simulink subsystem "Pumpstation_Controller"  (R2022b)
settings: Solver=VariableStepAuto  StartTime=0.0  StopTime=10.0  RelTol=1e-3
model mask{Speedlimit_Upper=95, Speedlimit_Lower=65, TotalPumps=3, Kp=0, Ki=0}
  mask prompts: Speedlimit_Upper "Upper limit on pump speed"; Speedlimit_Lower "Lower limit on pump speed"; TotalPumps "Total number of pumps"
libraries: slpidlib x1
settings Model: Creator=Fie  LastModifiedBy=pppc

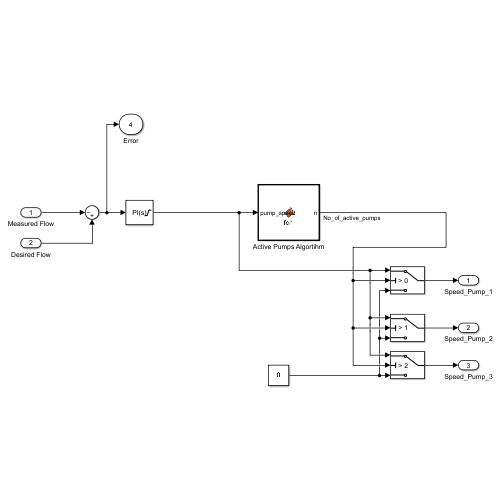
[thumbnail: Simulink's stored preview of the top-level diagram]
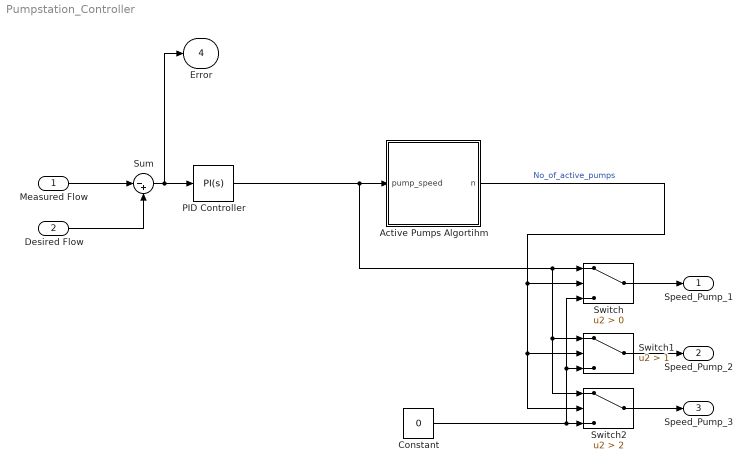
== system Pumpstation_Controller ==
  Measured Flow : Inport
  Desired Flow : Inport  Port=2
  Active Pumps Algortihm : MATLAB Function  TreatAsAtomicUnit=on  SystemSampleTime=10
  Constant : Constant  Value=0
  PID Controller : slpidlib/PID Controller  Controller=PI  Form=Parallel  TimeDomain=Continuous-time  UseExternalTs=off  SampleTime=-1  IntegratorMethod=Forward Euler  FilterMethod=Forward Euler  ControllerParametersSource=internal  P=Kp  I=Ki  UseKiTs=off  D=0  N=100  UseFilter=on  TunerSelectOption=Transfer Function Based (PID Tuner App)  InitialConditionSource=internal  InitialConditionForIntegrator=40  InitialConditionForFilter=0  DifferentiatorICPrevScaledInput=0  ExternalReset=none  TrackingMode=off  Kt=1  LimitOutput=on  SatLimitsSource=internal  UpperSaturationLimit=100  LowerSaturationLimit=0  LinearizeAsGain=on  AntiWindupMode=back-calculation  Kb=1  LimitIntegrator=off  UpperIntegratorSaturationLimit=inf  LowerIntegratorSaturationLimit=-inf  POutMin=[]  POutMax=[]  IOutMin=[]  IOutMax=[]  DOutMin=[]  DOutMax=[]  NOutMin=[]  NOutMax=[]  SumOutMin=[]  SumOutMax=[]  SaturationOutMin=[]  SaturationOutMax=[]  PParamMin=[]  PParamMax=[]  IParamMin=[]  IParamMax=[]  DParamMin=[]  DParamMax=[]  NParamMin=[]  NParamMax=[]  KbParamMin=[]  KbParamMax=[]  KtParamMin=[]  KtParamMax=[]  KbOutMin=[]  KbOutMax=[]  KtOutMin=[]  KtOutMax=[]  IntegratorOutMin=[]  IntegratorOutMax=[]  FilterOutMin=[]  FilterOutMax=[]  SumI1OutMin=[]  SumI1OutMax=[]  SumI2OutMin=[]  SumI2OutMax=[]  SumI3OutMin=[]  SumI3OutMax=[]  SumI4OutMin=[]  SumI4OutMax=[]  SumDOutMin=[]  SumDOutMax=[]  DifferentiatorOutMin=[]  DifferentiatorOutMax=[]  FilterDiffOutCoefMin=[]  FilterDiffOutCoefMax=[]  ReciprocalOutMin=[]  ReciprocalOutMax=[]  SumDenOutMin=[]  SumDenOutMax=[]  SumNumOutMin=[]  SumNumOutMax=[]  DivideOutMin=[]  DivideOutMax=[]  UdiffTsProdOutMin=[]  UdiffTsProdOutMax=[]  NTsProdOutMin=[]  NTsProdOutMax=[]  UintegralTsProdOutMin=[]  UintegralTsProdOutMax=[]  UngainTsProdOutMin=[]  UngainTsProdOutMax=[]  ClampingZeroOutDataTypeStr=Inherit: Inherit via back propagation  ClampingZeroOutMin=[]  ClampingZeroOutMax=[]  FilterDenConstantOutDataTypeStr=Inherit: Inherit via back propagation  FilterDenConstantOutMin=[]  FilterDenConstantOutMax=[]  PCopyOutDataTypeStr=Inherit: Inherit via back propagation  PCopyOutMin=[]  PCopyOutMax=[]  NCopyOutDataTypeStr=Inherit: Inherit via back propagation  NCopyOutMin=[]  NCopyOutMax=[]  IntegratorContinuousStateAttributes=''  IntegratorStateMustResolveToSignalObject=off  IntegratorRTWStateStorageClass=Auto  FilterContinuousStateAttributes=''  FilterStateMustResolveToSignalObject=off  FilterRTWStateStorageClass=Auto  ParallelPVariant=InternalParameters  IdealPVariant=Disabled  IVariant=InternalParameters  DVariant=Disabled  IntegratorVariant=Continuous  SatVariant=Enabled  AWVariant=BackCalculation  PCopyVariant=Disabled  TRVariant=Disabled  FdbkBlocksVariant=Forward  IdealPFdbkVariant=Disabled  SatFdbkVariant=Disabled  DerivativeFilterVariant=Disabled  NVariant=Disabled  NCopyVariant=Disabled_SignalSpec  FilterICVariant=Disabled  IntegratorICVariant=InternalICs  ExternalResetVariant=Disabled  TRSumVariant=Passthrough  SumFdbkVariant=Disabled  SumVariant=Sum_PI  TsampFilterVariant=InternalTs  TsampNgainVariant=Passthrough  TsampIntegralVariant=Passthrough  ExternalSaturationOutDataTypeStr=Inherit: Same as second input
  Sum : Sum  Inputs=|-+
  Switch : Switch  Criteria=u2 > Threshold  SaturateOnIntegerOverflow=off  InputSameDT=off
  Switch1 : Switch  Criteria=u2 > Threshold  Threshold=1  SaturateOnIntegerOverflow=off  InputSameDT=off
  Switch2 : Switch  Criteria=u2 > Threshold  Threshold=2  SaturateOnIntegerOverflow=off  InputSameDT=off
  Speed_Pump_1 : Outport
  Speed_Pump_2 : Outport  Port=2
  Speed_Pump_3 : Outport  Port=3
  Error : Outport  Port=4
  wires:
  Active Pumps Algortihm/1(n) -> Switch/2, Switch1/2, Switch2/2  "No_of_active_pumps"
  Constant/1 -> Switch2/3, Switch1/3, Switch/3
  Switch1/1 -> Speed_Pump_2/1
  Switch2/1 -> Speed_Pump_3/1
  Desired Flow/1 -> Sum/2
  Measured Flow/1 -> Sum/1
  Sum/1 -> PID Controller/1, Error/1
  Switch/1 -> Speed_Pump_1/1
  PID Controller/1 -> Switch/1, Switch1/1, Switch2/1, Active Pumps Algortihm/1(pump_speed)

== matlab function Pumpstation_Controller/Active Pumps Algortihm ==
  data: pump_speed input; n output; Speedlimit_Upper parameter; Speedlimit_Lower parameter; TotalPumps parameter
function n = fcn(pump_speed, Speedlimit_Upper, Speedlimit_Lower, TotalPumps)

persistent active_pumps

if isempty(active_pumps)
    active_pumps = 1;
end 


if pump_speed > Speedlimit_Upper 

    active_pumps = min(active_pumps+1, TotalPumps);

elseif pump_speed < Speedlimit_Lower

    active_pumps = max(active_pumps-1, 1);

end

n = active_pumps;
